simulink library "mcp2515lib"  (R2018b)
settings: Solver=VariableStepAuto  StartTime=0.0  StopTime=10.0  RelTol=1e-3  EnableMultiTasking=on
libraries: $bdroot x33, simulink x26, arduinolib x9, raspberrypilib x9
(part 2 of 2)

== system mcp2515lib/CAN application/CANreceive CE1/readRxBuffer/getDLC ==
  RxBx : Inport
  Bitwise Operator : simulink/Logic and Bit Operations/Bitwise Operator  logicop=AND  UseBitMask=off  NumInputPorts=2  BitMask=bin2dec('11011001')  BitMaskRealWorld=Stored Integer
  MCP_DLC_MASK : Constant  Value=hex2dec('0F')  OutDataTypeStr=uint8
  RxDLC : Selector  IndexMode=Zero-based  InputPortWidth=13  IndexOptions=Index vector (dialog)  Indices=4  OutputSizes=1
  CAN_dlc : Outport
  wires:
  MCP_DLC_MASK/1 -> Bitwise Operator/2
  RxDLC/1 -> Bitwise Operator/1
  RxBx/1 -> RxDLC/1
  Bitwise Operator/1 -> CAN_dlc/1

== system mcp2515lib/CAN application/CANreceive CE1/readRxBuffer/getData ==
  RxBx : Inport
  RxData : Selector  IndexMode=Zero-based  InputPortWidth=13  IndexOptions=Index vector (dialog)  Indices=[5:12]  OutputSizes=1
  CAN_data : Outport
  wires:
  RxData/1 -> CAN_data/1
  RxBx/1 -> RxData/1

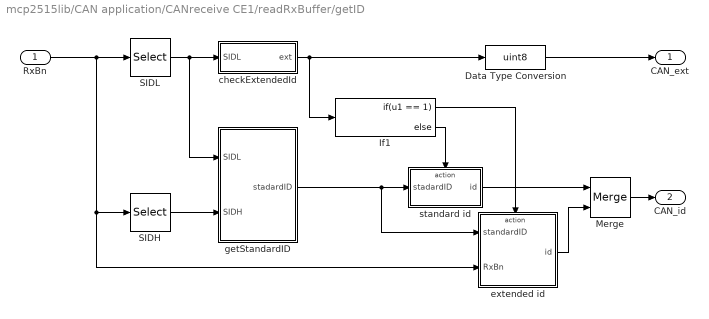
== system mcp2515lib/CAN application/CANreceive CE1/readRxBuffer/getID ==
  RxBn : Inport
  Data Type Conversion : DataTypeConversion  OutDataTypeStr=uint8  RndMeth=Simplest
  If1 : If  IfExpression=u1 == 1
  Merge : Merge
  SIDH : Selector  IndexMode=Zero-based  InputPortWidth=13  IndexOptions=Index vector (dialog)  Indices=0  OutputSizes=1
  SIDL : Selector  IndexMode=Zero-based  InputPortWidth=13  IndexOptions=Index vector (dialog)  Indices=1  OutputSizes=1
  checkExtendedId : Subsystem
  extended id : Subsystem  TreatAsAtomicUnit=on
      settings: RTWSystemCode=Inline
  getStandardID : Subsystem
  standard id : Subsystem  TreatAsAtomicUnit=on
      settings: RTWSystemCode=Inline
  CAN_ext : Outport
  CAN_id : Outport  Port=2
  wires:
  Data Type Conversion/1 -> CAN_ext/1
  checkExtendedId/1(ext) -> If1/1, Data Type Conversion/1
  SIDH/1 -> getStandardID/2(SIDH)
  SIDL/1 -> checkExtendedId/1(SIDL), getStandardID/1(SIDL)
  getStandardID/1(stadardID) -> extended id/1(standardID), standard id/1(stadardID)
  RxBn/1 -> SIDL/1, SIDH/1, extended id/2(RxBn)
  If1/1 -> extended id/Action
  If1/2 -> standard id/Action
  Merge/1 -> CAN_id/1
  extended id/1(id) -> Merge/2
  standard id/1(id) -> Merge/1

== system mcp2515lib/CAN application/CANtransmit/check TxB0/mcp2515_readRegister ==
  In : Inport
  address : Inport  Port=2  OutDataTypeStr=uint8
  Constant : Constant  Value=0  OutDataTypeStr=uint8
  MCP_READ : Constant  Value=3  OutDataTypeStr=uint8
  SPI driver : $bdroot/CAN application/mcp2515 driver/SPI driver  SystemSampleTime=-1
  Selector : Selector  IndexMode=Zero-based  InputPortWidth=3  IndexOptions=Index vector (dialog)  Indices=2  OutputSizes=1
  Vector Concatenate : Concatenate  NumInputs=3
  Out : Outport
  SPI_data : Outport  Port=2
  wires:
  Vector Concatenate/1 -> SPI driver/1
  Selector/1 -> SPI_data/1
  MCP_READ/1 -> Vector Concatenate/1
  In/1 -> Out/1
  Constant/1 -> Vector Concatenate/3
  address/1 -> Vector Concatenate/2
  SPI driver/1 -> Selector/1

== system mcp2515lib/CAN application/CANtransmit/load Tx data/mcp2515_writeTxBuffer ==
  In : Inport
  cmd_load_tx_buff : Inport  Port=2
  data_tx_buff : Inport  Port=3
  SPI driver : $bdroot/CAN application/mcp2515 driver/SPI driver  SystemSampleTime=-1
  Selector1 : Selector  IndexMode=Zero-based  InputPortWidth=14  IndexOptions=Index vector (dialog)  Indices=0  OutputSizes=1
  Temporary buffer : DataStoreWrite  DataStoreName=temp_1byte
  Vector Concatenate : Concatenate
  Out : Outport
  wires:
  Vector Concatenate/1 -> SPI driver/1
  Selector1/1 -> Temporary buffer/1
  cmd_load_tx_buff/1 -> Vector Concatenate/1
  data_tx_buff/1 -> Vector Concatenate/2
  SPI driver/1 -> Selector1/1
  In/1 -> Out/1

== system mcp2515lib/CAN application/CANtransmit/load Tx data/setID ==
  ext : Inport
  id : Inport  Port=2
  Extended ID : Subsystem  TreatAsAtomicUnit=on
  If : If
  Merge : Merge
  Standard ID : Subsystem  TreatAsAtomicUnit=on
  TxBn_ID : Outport
  wires:
  id/1 -> Standard ID/1(id), Extended ID/1(id)
  Merge/1 -> TxBn_ID/1
  Standard ID/1(TxBn_ID) -> Merge/1
  Extended ID/1(TxBn_ID) -> Merge/2
  If/2 -> Standard ID/Action
  If/1 -> Extended ID/Action
  ext/1 -> If/1

== system mcp2515lib/CAN application/CANtransmit/send TxB0/mcp2515_writeRegister ==
  In : Inport
  address : Inport  Port=2  OutDataTypeStr=uint8
  value : Inport  Port=3  OutDataTypeStr=uint8
  MCP_WRITE : Constant  Value=2  OutDataTypeStr=uint8
  SPI driver : $bdroot/CAN application/mcp2515 driver/SPI driver  SystemSampleTime=-1
  Selector : Selector  IndexMode=Zero-based  InputPortWidth=3  IndexOptions=Index vector (dialog)  Indices=0  OutputSizes=1
  Temporary buffer : DataStoreWrite  DataStoreName=temp_1byte
  Vector Concatenate : Concatenate  NumInputs=3
  Out : Outport
  wires:
  MCP_WRITE/1 -> Vector Concatenate/1
  address/1 -> Vector Concatenate/2
  value/1 -> Vector Concatenate/3
  Vector Concatenate/1 -> SPI driver/1
  In/1 -> Out/1
  Selector/1 -> Temporary buffer/1
  SPI driver/1 -> Selector/1

== system mcp2515lib/CAN application/CANtransmit CE1/load Tx data/setID ==
  ext : Inport
  id : Inport  Port=2
  Extended ID : Subsystem  TreatAsAtomicUnit=on
  If : If
  Merge : Merge
  Standard ID : Subsystem  TreatAsAtomicUnit=on
  TxBn_ID : Outport
  wires:
  id/1 -> Standard ID/1(id), Extended ID/1(id)
  Merge/1 -> TxBn_ID/1
  Standard ID/1(TxBn_ID) -> Merge/1
  Extended ID/1(TxBn_ID) -> Merge/2
  If/2 -> Standard ID/Action
  If/1 -> Extended ID/Action
  ext/1 -> If/1

== system mcp2515lib/CAN application/mcp2515 driver/SPI driver/Arduino ==
  SPIdata_In : Inport
  SPI WriteRead : arduinolib/SPI WriteRead  slaveSelectPin_=CSpin  blockPlatform=arduino
      settings: SourceProductName=Simulink Support Package for Arduino Hardware  SourceProductBaseCode=ARDUINO
  SPIdata_Out : Outport
  wires:
  SPIdata_In/1 -> SPI WriteRead/1
  SPI WriteRead/1 -> SPIdata_Out/1

== system mcp2515lib/CAN application/mcp2515 driver/SPI driver/Rapberry Pi ==
  SPIdata_In : Inport
  SPI Master Transfer : raspberrypilib/SPI Master Transfer  BoardProperty=Pi 3 Model B+  SPIModule=uint32(0)  Mode=Master  BusSpeed=1000000  Pin=SPI0_CE0  FirstBitToTransfer=Most significant bit (MSB)  ClockMode=0  BlockFunction=Transfer  RegisterAddress=0  OutputDataType=int8  OutputDataLength=1
      settings: SourceProductName=Simulink Support Package for Raspberry Pi Hardware  SourceProductBaseCode=RASPPI
  SPIdata_Out : Outport
  wires:
  SPIdata_In/1 -> SPI Master Transfer/1
  SPI Master Transfer/1 -> SPIdata_Out/1

== system mcp2515lib/CAN application/mcp2515 driver CE1/SPI driver/Arduino ==
  SPIdata_In : Inport
  SPI WriteRead : arduinolib/SPI WriteRead  slaveSelectPin_=CSpin  blockPlatform=arduino
      settings: SourceProductName=Simulink Support Package for Arduino Hardware  SourceProductBaseCode=ARDUINO
  SPIdata_Out : Outport
  wires:
  SPI WriteRead/1 -> SPIdata_Out/1
  SPIdata_In/1 -> SPI WriteRead/1

== system mcp2515lib/CAN application/mcp2515 driver CE1/SPI driver/Rapberry Pi ==
  SPIdata_In : Inport
  SPI Master Transfer : raspberrypilib/SPI Master Transfer  BoardProperty=Pi 3 Model B+  SPIModule=uint32(0)  Mode=Master  BusSpeed=1000000  Pin=SPI0_CE1  FirstBitToTransfer=Most significant bit (MSB)  ClockMode=0  BlockFunction=Transfer  RegisterAddress=0  OutputDataType=int8  OutputDataLength=1
      settings: SourceProductName=Simulink Support Package for Raspberry Pi Hardware  SourceProductBaseCode=RASPPI
  SPIdata_Out : Outport
  wires:
  SPI Master Transfer/1 -> SPIdata_Out/1
  SPIdata_In/1 -> SPI Master Transfer/1

== system mcp2515lib/CAN application/mcp2515 driver CE1/mcp2515_modifyRegister/SPI driver ==
  SPIdata_In : Inport
  Arduino : Subsystem  TreatAsAtomicUnit=on  VariantControl=Hardware == 1
  Rapberry Pi : Subsystem  TreatAsAtomicUnit=on  VariantControl=Hardware == 2
  SPIdata_Out : Outport

== system mcp2515lib/CAN application/mcp2515 driver CE1/mcp2515_readRegister/SPI driver ==
  SPIdata_In : Inport
  Arduino : Subsystem  TreatAsAtomicUnit=on  VariantControl=Hardware == 1
  Rapberry Pi : Subsystem  TreatAsAtomicUnit=on  VariantControl=Hardware == 2
  SPIdata_Out : Outport

== system mcp2515lib/CAN application/mcp2515 driver CE1/mcp2515_readRxBuffer/SPI driver ==
  SPIdata_In : Inport
  Arduino : Subsystem  TreatAsAtomicUnit=on  VariantControl=Hardware == 1
  Rapberry Pi : Subsystem  TreatAsAtomicUnit=on  VariantControl=Hardware == 2
  SPIdata_Out : Outport

== system mcp2515lib/CAN application/mcp2515 driver CE1/mcp2515_read_RX_STATUS/SPI driver ==
  SPIdata_In : Inport
  Arduino : Subsystem  TreatAsAtomicUnit=on  VariantControl=Hardware == 1
  Rapberry Pi : Subsystem  TreatAsAtomicUnit=on  VariantControl=Hardware == 2
  SPIdata_Out : Outport

== system mcp2515lib/CAN application/mcp2515 driver CE1/mcp2515_reset/SPI driver ==
  SPIdata_In : Inport
  Arduino : Subsystem  TreatAsAtomicUnit=on  VariantControl=Hardware == 1
  Rapberry Pi : Subsystem  TreatAsAtomicUnit=on  VariantControl=Hardware == 2
  SPIdata_Out : Outport

== system mcp2515lib/CAN application/mcp2515 driver CE1/mcp2515_writeRegister/SPI driver ==
  SPIdata_In : Inport
  Arduino : Subsystem  TreatAsAtomicUnit=on  VariantControl=Hardware == 1
  Rapberry Pi : Subsystem  TreatAsAtomicUnit=on  VariantControl=Hardware == 2
  SPIdata_Out : Outport

== system mcp2515lib/CAN application/mcp2515 driver CE1/mcp2515_writeTxBuffer/SPI driver ==
  SPIdata_In : Inport
  Arduino : Subsystem  TreatAsAtomicUnit=on  VariantControl=Hardware == 1
  Rapberry Pi : Subsystem  TreatAsAtomicUnit=on  VariantControl=Hardware == 2
  SPIdata_Out : Outport

== system mcp2515lib/CAN application/CANbegin/setup/changeCANmode(config)/mcp2515_modifyRegister ==
  In : Inport
  address : Inport  Port=2
  mask : Inport  Port=3
  data : Inport  Port=4
  MCP_BITMOD : Constant  Value=5  OutDataTypeStr=uint8
  SPI driver : $bdroot/CAN application/mcp2515 driver/SPI driver  SystemSampleTime=-1
  Selector : Selector  IndexMode=Zero-based  InputPortWidth=4  IndexOptions=Index vector (dialog)  Indices=0  OutputSizes=1
  Temporary buffer : DataStoreWrite  DataStoreName=temp_1byte
  Vector Concatenate : Concatenate  NumInputs=4
  Out : Outport
  wires:
  Vector Concatenate/1 -> SPI driver/1
  Selector/1 -> Temporary buffer/1
  In/1 -> Out/1
  MCP_BITMOD/1 -> Vector Concatenate/1
  mask/1 -> Vector Concatenate/3
  address/1 -> Vector Concatenate/2
  data/1 -> Vector Concatenate/4
  SPI driver/1 -> Selector/1

== system mcp2515lib/CAN application/CANbegin/setup/changeCANmode(normal)/mcp2515_modifyRegister ==
  In : Inport
  address : Inport  Port=2
  mask : Inport  Port=3
  data : Inport  Port=4
  MCP_BITMOD : Constant  Value=5  OutDataTypeStr=uint8
  SPI driver : $bdroot/CAN application/mcp2515 driver/SPI driver  SystemSampleTime=-1
  Selector : Selector  IndexMode=Zero-based  InputPortWidth=4  IndexOptions=Index vector (dialog)  Indices=0  OutputSizes=1
  Temporary buffer : DataStoreWrite  DataStoreName=temp_1byte
  Vector Concatenate : Concatenate  NumInputs=4
  Out : Outport
  wires:
  Vector Concatenate/1 -> SPI driver/1
  Selector/1 -> Temporary buffer/1
  In/1 -> Out/1
  MCP_BITMOD/1 -> Vector Concatenate/1
  mask/1 -> Vector Concatenate/3
  address/1 -> Vector Concatenate/2
  data/1 -> Vector Concatenate/4
  SPI driver/1 -> Selector/1

== system mcp2515lib/CAN application/CANbegin/setup/setCANRxBuffer/mcp2515_writeRegister ==
  In : Inport
  address : Inport  Port=2  OutDataTypeStr=uint8
  value : Inport  Port=3  OutDataTypeStr=uint8
  MCP_WRITE : Constant  Value=2  OutDataTypeStr=uint8
  SPI driver : $bdroot/CAN application/mcp2515 driver/SPI driver  SystemSampleTime=-1
  Selector : Selector  IndexMode=Zero-based  InputPortWidth=3  IndexOptions=Index vector (dialog)  Indices=0  OutputSizes=1
  Temporary buffer : DataStoreWrite  DataStoreName=temp_1byte
  Vector Concatenate : Concatenate  NumInputs=3
  Out : Outport
  wires:
  MCP_WRITE/1 -> Vector Concatenate/1
  address/1 -> Vector Concatenate/2
  value/1 -> Vector Concatenate/3
  Vector Concatenate/1 -> SPI driver/1
  In/1 -> Out/1
  Selector/1 -> Temporary buffer/1
  SPI driver/1 -> Selector/1

== system mcp2515lib/CAN application/CANbegin/setup/setCANRxBuffer/mcp2515_writeRegister1 ==
  In : Inport
  address : Inport  Port=2  OutDataTypeStr=uint8
  value : Inport  Port=3  OutDataTypeStr=uint8
  MCP_WRITE : Constant  Value=2  OutDataTypeStr=uint8
  SPI driver : $bdroot/CAN application/mcp2515 driver/SPI driver  SystemSampleTime=-1
  Selector : Selector  IndexMode=Zero-based  InputPortWidth=3  IndexOptions=Index vector (dialog)  Indices=0  OutputSizes=1
  Temporary buffer : DataStoreWrite  DataStoreName=temp_1byte
  Vector Concatenate : Concatenate  NumInputs=3
  Out : Outport
  wires:
  MCP_WRITE/1 -> Vector Concatenate/1
  address/1 -> Vector Concatenate/2
  value/1 -> Vector Concatenate/3
  Vector Concatenate/1 -> SPI driver/1
  In/1 -> Out/1
  Selector/1 -> Temporary buffer/1
  SPI driver/1 -> Selector/1

== system mcp2515lib/CAN application/CANbegin/setup/setCANspeed/mcp2515_writeRegister1 ==
  In : Inport
  address : Inport  Port=2  OutDataTypeStr=uint8
  value : Inport  Port=3  OutDataTypeStr=uint8
  MCP_WRITE : Constant  Value=2  OutDataTypeStr=uint8
  SPI driver : $bdroot/CAN application/mcp2515 driver/SPI driver  SystemSampleTime=-1
  Selector : Selector  IndexMode=Zero-based  InputPortWidth=3  IndexOptions=Index vector (dialog)  Indices=0  OutputSizes=1
  Temporary buffer : DataStoreWrite  DataStoreName=temp_1byte
  Vector Concatenate : Concatenate  NumInputs=3
  Out : Outport
  wires:
  MCP_WRITE/1 -> Vector Concatenate/1
  address/1 -> Vector Concatenate/2
  value/1 -> Vector Concatenate/3
  Vector Concatenate/1 -> SPI driver/1
  In/1 -> Out/1
  Selector/1 -> Temporary buffer/1
  SPI driver/1 -> Selector/1

== system mcp2515lib/CAN application/CANbegin/setup/setCANspeed/mcp2515_writeRegister2 ==
  In : Inport
  address : Inport  Port=2  OutDataTypeStr=uint8
  value : Inport  Port=3  OutDataTypeStr=uint8
  MCP_WRITE : Constant  Value=2  OutDataTypeStr=uint8
  SPI driver : $bdroot/CAN application/mcp2515 driver/SPI driver  SystemSampleTime=-1
  Selector : Selector  IndexMode=Zero-based  InputPortWidth=3  IndexOptions=Index vector (dialog)  Indices=0  OutputSizes=1
  Temporary buffer : DataStoreWrite  DataStoreName=temp_1byte
  Vector Concatenate : Concatenate  NumInputs=3
  Out : Outport
  wires:
  MCP_WRITE/1 -> Vector Concatenate/1
  address/1 -> Vector Concatenate/2
  value/1 -> Vector Concatenate/3
  Vector Concatenate/1 -> SPI driver/1
  In/1 -> Out/1
  Selector/1 -> Temporary buffer/1
  SPI driver/1 -> Selector/1

== system mcp2515lib/CAN application/CANbegin/setup/setCANspeed/mcp2515_writeRegister3 ==
  In : Inport
  address : Inport  Port=2  OutDataTypeStr=uint8
  value : Inport  Port=3  OutDataTypeStr=uint8
  MCP_WRITE : Constant  Value=2  OutDataTypeStr=uint8
  SPI driver : $bdroot/CAN application/mcp2515 driver/SPI driver  SystemSampleTime=-1
  Selector : Selector  IndexMode=Zero-based  InputPortWidth=3  IndexOptions=Index vector (dialog)  Indices=0  OutputSizes=1
  Temporary buffer : DataStoreWrite  DataStoreName=temp_1byte
  Vector Concatenate : Concatenate  NumInputs=3
  Out : Outport
  wires:
  MCP_WRITE/1 -> Vector Concatenate/1
  address/1 -> Vector Concatenate/2
  value/1 -> Vector Concatenate/3
  Vector Concatenate/1 -> SPI driver/1
  In/1 -> Out/1
  Selector/1 -> Temporary buffer/1
  SPI driver/1 -> Selector/1

== system mcp2515lib/CAN application/CANreceive/readRxBuffer/getID/checkExtendedId ==
  SIDL : Inport
  Bitmask_EXIDE : simulink/Logic and Bit Operations/Bitwise Operator  logicop=AND  UseBitMask=on  BitMask=bin2dec('00001000')  BitMaskRealWorld=Stored Integer
  MCP_TXB_EXIDE_M : Constant  Value=hex2dec('08')  OutDataTypeStr=uint8
  Relational Operator : RelationalOperator  Operator===  OutDataTypeStr=boolean  RndMeth=Nearest
  ext : Outport
  wires:
  SIDL/1 -> Bitmask_EXIDE/1
  Bitmask_EXIDE/1 -> Relational Operator/2
  MCP_TXB_EXIDE_M/1 -> Relational Operator/1
  Relational Operator/1 -> ext/1

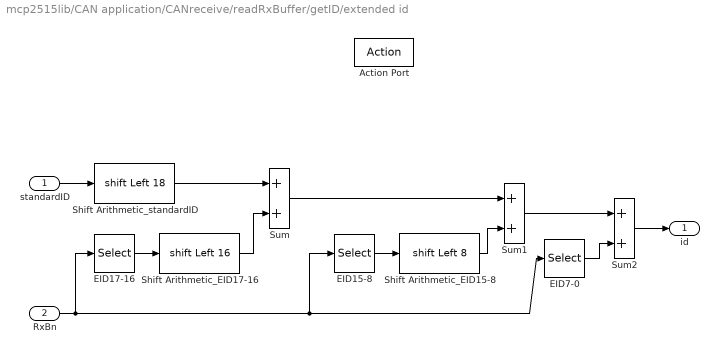
== system mcp2515lib/CAN application/CANreceive/readRxBuffer/getID/extended id ==
  standardID : Inport
  RxBn : Inport  Port=2
  Action Port : ActionPort
  EID15-8 : Selector  IndexMode=Zero-based  InputPortWidth=13  IndexOptions=Index vector (dialog)  Indices=2  OutputSizes=1
  EID17-16 : Selector  IndexMode=Zero-based  InputPortWidth=13  IndexOptions=Index vector (dialog)  Indices=1  OutputSizes=1
  EID7-0 : Selector  IndexMode=Zero-based  InputPortWidth=13  IndexOptions=Index vector (dialog)  Indices=3  OutputSizes=1
  Shift Arithmetic_EID15-8 : ArithShift  BitShiftNumber=8  BitShiftDirection=Left
  Shift Arithmetic_EID17-16 : ArithShift  BitShiftNumber=16  BitShiftDirection=Left
  Shift Arithmetic_standardID : ArithShift  BitShiftNumber=18  BitShiftDirection=Left
  Sum : Sum
  Sum1 : Sum
  Sum2 : Sum
  id : Outport
  wires:
  EID7-0/1 -> Sum2/2
  RxBn/1 -> EID17-16/1, EID15-8/1, EID7-0/1
  Sum1/1 -> Sum2/1
  EID15-8/1 -> Shift Arithmetic_EID15-8/1
  Shift Arithmetic_EID15-8/1 -> Sum1/2
  Sum/1 -> Sum1/1
  Shift Arithmetic_EID17-16/1 -> Sum/2
  EID17-16/1 -> Shift Arithmetic_EID17-16/1
  Shift Arithmetic_standardID/1 -> Sum/1
  standardID/1 -> Shift Arithmetic_standardID/1
  Sum2/1 -> id/1

== system mcp2515lib/CAN application/CANreceive/readRxBuffer/getID/getStandardID ==
  SIDL : Inport
  SIDH : Inport  Port=2
  Bitmask_SID2-0 : simulink/Logic and Bit Operations/Bitwise Operator  logicop=AND  UseBitMask=on  BitMask=bin2dec('11100000')  BitMaskRealWorld=Stored Integer
  Data Type Conversion : DataTypeConversion  OutDataTypeStr=uint32
  Shift Arithmetic_SID10-3 : ArithShift  BitShiftNumber=3  BitShiftDirection=Left
  Shift Arithmetic_SID2-0 : ArithShift  BitShiftNumber=5  BitShiftDirection=Right
  Sum1 : Sum
  stadardID : Outport
  wires:
  Data Type Conversion/1 -> Shift Arithmetic_SID10-3/1
  Bitmask_SID2-0/1 -> Shift Arithmetic_SID2-0/1
  SIDH/1 -> Data Type Conversion/1
  SIDL/1 -> Bitmask_SID2-0/1
  Shift Arithmetic_SID10-3/1 -> Sum1/2
  Shift Arithmetic_SID2-0/1 -> Sum1/1
  Sum1/1 -> stadardID/1

== system mcp2515lib/CAN application/CANreceive/readRxBuffer/getID/standard id ==
  stadardID : Inport
  Action Port : ActionPort
  id : Outport
  wires:
  stadardID/1 -> id/1

== system mcp2515lib/CAN application/CANreceive CE1/readRxBuffer/getID/checkExtendedId ==
  SIDL : Inport
  Bitmask_EXIDE : simulink/Logic and Bit Operations/Bitwise Operator  logicop=AND  UseBitMask=on  BitMask=bin2dec('00001000')  BitMaskRealWorld=Stored Integer
  MCP_TXB_EXIDE_M : Constant  Value=hex2dec('08')  OutDataTypeStr=uint8
  Relational Operator : RelationalOperator  Operator===  OutDataTypeStr=boolean  RndMeth=Nearest
  ext : Outport
  wires:
  SIDL/1 -> Bitmask_EXIDE/1
  Bitmask_EXIDE/1 -> Relational Operator/2
  MCP_TXB_EXIDE_M/1 -> Relational Operator/1
  Relational Operator/1 -> ext/1

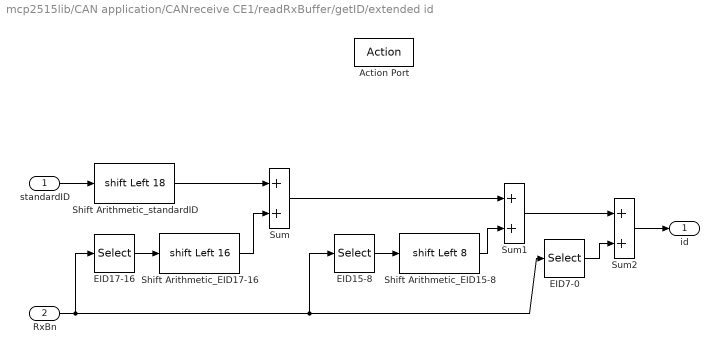
== system mcp2515lib/CAN application/CANreceive CE1/readRxBuffer/getID/extended id ==
  standardID : Inport
  RxBn : Inport  Port=2
  Action Port : ActionPort
  EID15-8 : Selector  IndexMode=Zero-based  InputPortWidth=13  IndexOptions=Index vector (dialog)  Indices=2  OutputSizes=1
  EID17-16 : Selector  IndexMode=Zero-based  InputPortWidth=13  IndexOptions=Index vector (dialog)  Indices=1  OutputSizes=1
  EID7-0 : Selector  IndexMode=Zero-based  InputPortWidth=13  IndexOptions=Index vector (dialog)  Indices=3  OutputSizes=1
  Shift Arithmetic_EID15-8 : ArithShift  BitShiftNumber=8  BitShiftDirection=Left
  Shift Arithmetic_EID17-16 : ArithShift  BitShiftNumber=16  BitShiftDirection=Left
  Shift Arithmetic_standardID : ArithShift  BitShiftNumber=18  BitShiftDirection=Left
  Sum : Sum
  Sum1 : Sum
  Sum2 : Sum
  id : Outport
  wires:
  EID7-0/1 -> Sum2/2
  RxBn/1 -> EID17-16/1, EID15-8/1, EID7-0/1
  Sum1/1 -> Sum2/1
  EID15-8/1 -> Shift Arithmetic_EID15-8/1
  Shift Arithmetic_EID15-8/1 -> Sum1/2
  Sum/1 -> Sum1/1
  Shift Arithmetic_EID17-16/1 -> Sum/2
  EID17-16/1 -> Shift Arithmetic_EID17-16/1
  Shift Arithmetic_standardID/1 -> Sum/1
  standardID/1 -> Shift Arithmetic_standardID/1
  Sum2/1 -> id/1

== system mcp2515lib/CAN application/CANreceive CE1/readRxBuffer/getID/getStandardID ==
  SIDL : Inport
  SIDH : Inport  Port=2
  Bitmask_SID2-0 : simulink/Logic and Bit Operations/Bitwise Operator  logicop=AND  UseBitMask=on  BitMask=bin2dec('11100000')  BitMaskRealWorld=Stored Integer
  Data Type Conversion : DataTypeConversion  OutDataTypeStr=uint32
  Shift Arithmetic_SID10-3 : ArithShift  BitShiftNumber=3  BitShiftDirection=Left
  Shift Arithmetic_SID2-0 : ArithShift  BitShiftNumber=5  BitShiftDirection=Right
  Sum1 : Sum
  stadardID : Outport
  wires:
  Data Type Conversion/1 -> Shift Arithmetic_SID10-3/1
  Bitmask_SID2-0/1 -> Shift Arithmetic_SID2-0/1
  SIDH/1 -> Data Type Conversion/1
  SIDL/1 -> Bitmask_SID2-0/1
  Shift Arithmetic_SID10-3/1 -> Sum1/2
  Shift Arithmetic_SID2-0/1 -> Sum1/1
  Sum1/1 -> stadardID/1

== system mcp2515lib/CAN application/CANreceive CE1/readRxBuffer/getID/standard id ==
  stadardID : Inport
  Action Port : ActionPort
  id : Outport
  wires:
  stadardID/1 -> id/1

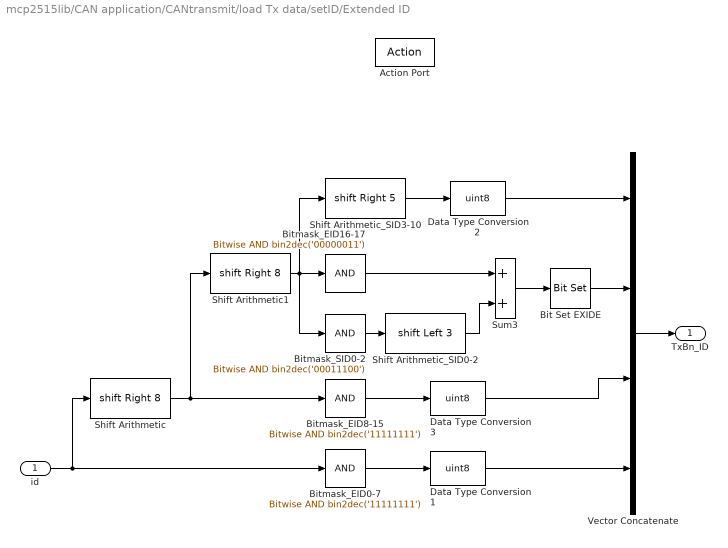
== system mcp2515lib/CAN application/CANtransmit/load Tx data/setID/Extended ID ==
  id : Inport
  Action Port : ActionPort
  Bit Set EXIDE : simulink/Logic and Bit Operations/Bit Set  iBit=3
      settings: SourceProductName=Simulink  SourceProductBaseCode=SL
  Bitmask_EID0-7 : simulink/Logic and Bit Operations/Bitwise Operator  logicop=AND  UseBitMask=on  BitMask=bin2dec('11111111')  BitMaskRealWorld=Stored Integer
  Bitmask_EID16-17 : simulink/Logic and Bit Operations/Bitwise Operator  logicop=AND  UseBitMask=on  BitMask=bin2dec('00000011')  BitMaskRealWorld=Stored Integer
  Bitmask_EID8-15 : simulink/Logic and Bit Operations/Bitwise Operator  logicop=AND  UseBitMask=on  BitMask=bin2dec('11111111')  BitMaskRealWorld=Stored Integer
  Bitmask_SID0-2 : simulink/Logic and Bit Operations/Bitwise Operator  logicop=AND  UseBitMask=on  BitMask=bin2dec('00011100')  BitMaskRealWorld=Stored Integer
  Data Type Conversion1 : DataTypeConversion  OutDataTypeStr=uint8  RndMeth=Simplest
  Data Type Conversion2 : DataTypeConversion  OutDataTypeStr=uint8  RndMeth=Simplest
  Data Type Conversion3 : DataTypeConversion  OutDataTypeStr=uint8  RndMeth=Simplest
  Shift Arithmetic : ArithShift  BitShiftNumber=8  BitShiftDirection=Right
  Shift Arithmetic1 : ArithShift  BitShiftNumber=8  BitShiftDirection=Right
  Shift Arithmetic_SID0-2 : ArithShift  BitShiftNumber=3  BitShiftDirection=Left
  Shift Arithmetic_SID3-10 : ArithShift  BitShiftNumber=5  BitShiftDirection=Right
  Sum3 : Sum  OutDataTypeStr=uint8
  Vector Concatenate : Concatenate  NumInputs=4
  TxBn_ID : Outport
  wires:
  Data Type Conversion2/1 -> Vector Concatenate/1
  Shift Arithmetic_SID3-10/1 -> Data Type Conversion2/1
  Bit Set EXIDE/1 -> Vector Concatenate/2
  Shift Arithmetic_SID0-2/1 -> Sum3/2
  Bitmask_SID0-2/1 -> Shift Arithmetic_SID0-2/1
  Bitmask_EID16-17/1 -> Sum3/1
  Sum3/1 -> Bit Set EXIDE/1
  Shift Arithmetic1/1 -> Bitmask_EID16-17/1, Bitmask_SID0-2/1, Shift Arithmetic_SID3-10/1
  Data Type Conversion3/1 -> Vector Concatenate/3
  Bitmask_EID8-15/1 -> Data Type Conversion3/1
  Shift Arithmetic/1 -> Bitmask_EID8-15/1, Shift Arithmetic1/1
  Data Type Conversion1/1 -> Vector Concatenate/4
  Bitmask_EID0-7/1 -> Data Type Conversion1/1
  id/1 -> Bitmask_EID0-7/1, Shift Arithmetic/1
  Vector Concatenate/1 -> TxBn_ID/1

== system mcp2515lib/CAN application/CANtransmit/load Tx data/setID/Standard ID ==
  id : Inport
  Action Port : ActionPort
  Vector Concatenate : Concatenate  NumInputs=4
  convert_ID : Subsystem  TreatAsAtomicUnit=on
  no data : Constant  Value=0  OutDataTypeStr=uint8
  TxBn_ID : Outport
  wires:
  convert_ID/1(SIDH) -> Vector Concatenate/1
  id/1 -> convert_ID/1(id)
  convert_ID/2(SIDL) -> Vector Concatenate/2
  no data/1 -> Vector Concatenate/4, Vector Concatenate/3
  Vector Concatenate/1 -> TxBn_ID/1

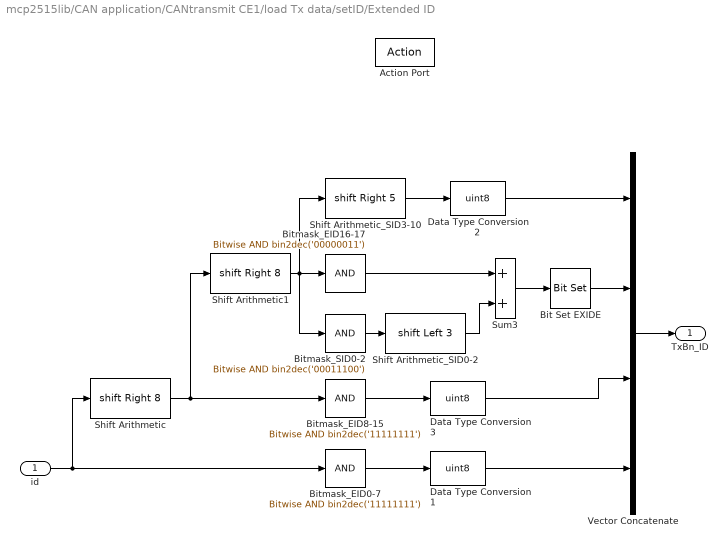
== system mcp2515lib/CAN application/CANtransmit CE1/load Tx data/setID/Extended ID ==
  id : Inport
  Action Port : ActionPort
  Bit Set EXIDE : simulink/Logic and Bit Operations/Bit Set  iBit=3
      settings: SourceProductName=Simulink  SourceProductBaseCode=SL
  Bitmask_EID0-7 : simulink/Logic and Bit Operations/Bitwise Operator  logicop=AND  UseBitMask=on  BitMask=bin2dec('11111111')  BitMaskRealWorld=Stored Integer
  Bitmask_EID16-17 : simulink/Logic and Bit Operations/Bitwise Operator  logicop=AND  UseBitMask=on  BitMask=bin2dec('00000011')  BitMaskRealWorld=Stored Integer
  Bitmask_EID8-15 : simulink/Logic and Bit Operations/Bitwise Operator  logicop=AND  UseBitMask=on  BitMask=bin2dec('11111111')  BitMaskRealWorld=Stored Integer
  Bitmask_SID0-2 : simulink/Logic and Bit Operations/Bitwise Operator  logicop=AND  UseBitMask=on  BitMask=bin2dec('00011100')  BitMaskRealWorld=Stored Integer
  Data Type Conversion1 : DataTypeConversion  OutDataTypeStr=uint8  RndMeth=Simplest
  Data Type Conversion2 : DataTypeConversion  OutDataTypeStr=uint8  RndMeth=Simplest
  Data Type Conversion3 : DataTypeConversion  OutDataTypeStr=uint8  RndMeth=Simplest
  Shift Arithmetic : ArithShift  BitShiftNumber=8  BitShiftDirection=Right
  Shift Arithmetic1 : ArithShift  BitShiftNumber=8  BitShiftDirection=Right
  Shift Arithmetic_SID0-2 : ArithShift  BitShiftNumber=3  BitShiftDirection=Left
  Shift Arithmetic_SID3-10 : ArithShift  BitShiftNumber=5  BitShiftDirection=Right
  Sum3 : Sum  OutDataTypeStr=uint8
  Vector Concatenate : Concatenate  NumInputs=4
  TxBn_ID : Outport
  wires:
  Data Type Conversion2/1 -> Vector Concatenate/1
  Shift Arithmetic_SID3-10/1 -> Data Type Conversion2/1
  Bit Set EXIDE/1 -> Vector Concatenate/2
  Shift Arithmetic_SID0-2/1 -> Sum3/2
  Bitmask_SID0-2/1 -> Shift Arithmetic_SID0-2/1
  Bitmask_EID16-17/1 -> Sum3/1
  Sum3/1 -> Bit Set EXIDE/1
  Shift Arithmetic1/1 -> Bitmask_EID16-17/1, Bitmask_SID0-2/1, Shift Arithmetic_SID3-10/1
  Data Type Conversion3/1 -> Vector Concatenate/3
  Bitmask_EID8-15/1 -> Data Type Conversion3/1
  Shift Arithmetic/1 -> Bitmask_EID8-15/1, Shift Arithmetic1/1
  Data Type Conversion1/1 -> Vector Concatenate/4
  Bitmask_EID0-7/1 -> Data Type Conversion1/1
  id/1 -> Bitmask_EID0-7/1, Shift Arithmetic/1
  Vector Concatenate/1 -> TxBn_ID/1

== system mcp2515lib/CAN application/CANtransmit CE1/load Tx data/setID/Standard ID ==
  id : Inport
  Action Port : ActionPort
  Vector Concatenate : Concatenate  NumInputs=4
  convert_ID : Subsystem  TreatAsAtomicUnit=on
  no data : Constant  Value=0  OutDataTypeStr=uint8
  TxBn_ID : Outport
  wires:
  convert_ID/1(SIDH) -> Vector Concatenate/1
  id/1 -> convert_ID/1(id)
  convert_ID/2(SIDL) -> Vector Concatenate/2
  no data/1 -> Vector Concatenate/4, Vector Concatenate/3
  Vector Concatenate/1 -> TxBn_ID/1

== system mcp2515lib/CAN application/mcp2515 driver CE1/mcp2515_modifyRegister/SPI driver/Arduino ==
  SPIdata_In : Inport
  SPI WriteRead : arduinolib/SPI WriteRead  slaveSelectPin_=CSpin  blockPlatform=arduino
      settings: SourceProductName=Simulink Support Package for Arduino Hardware  SourceProductBaseCode=ARDUINO
  SPIdata_Out : Outport
  wires:
  SPI WriteRead/1 -> SPIdata_Out/1
  SPIdata_In/1 -> SPI WriteRead/1

== system mcp2515lib/CAN application/mcp2515 driver CE1/mcp2515_modifyRegister/SPI driver/Rapberry Pi ==
  SPIdata_In : Inport
  SPI Master Transfer : raspberrypilib/SPI Master Transfer  BoardProperty=Pi 3 Model B+  SPIModule=uint32(0)  Mode=Master  BusSpeed=1000000  Pin=SPI0_CE1  FirstBitToTransfer=Most significant bit (MSB)  ClockMode=0  BlockFunction=Transfer  RegisterAddress=0  OutputDataType=int8  OutputDataLength=1
      settings: SourceProductName=Simulink Support Package for Raspberry Pi Hardware  SourceProductBaseCode=RASPPI
  SPIdata_Out : Outport
  wires:
  SPI Master Transfer/1 -> SPIdata_Out/1
  SPIdata_In/1 -> SPI Master Transfer/1

== system mcp2515lib/CAN application/mcp2515 driver CE1/mcp2515_readRegister/SPI driver/Arduino ==
  SPIdata_In : Inport
  SPI WriteRead : arduinolib/SPI WriteRead  slaveSelectPin_=CSpin  blockPlatform=arduino
      settings: SourceProductName=Simulink Support Package for Arduino Hardware  SourceProductBaseCode=ARDUINO
  SPIdata_Out : Outport
  wires:
  SPI WriteRead/1 -> SPIdata_Out/1
  SPIdata_In/1 -> SPI WriteRead/1

== system mcp2515lib/CAN application/mcp2515 driver CE1/mcp2515_readRegister/SPI driver/Rapberry Pi ==
  SPIdata_In : Inport
  SPI Master Transfer : raspberrypilib/SPI Master Transfer  BoardProperty=Pi 3 Model B+  SPIModule=uint32(0)  Mode=Master  BusSpeed=1000000  Pin=SPI0_CE1  FirstBitToTransfer=Most significant bit (MSB)  ClockMode=0  BlockFunction=Transfer  RegisterAddress=0  OutputDataType=int8  OutputDataLength=1
      settings: SourceProductName=Simulink Support Package for Raspberry Pi Hardware  SourceProductBaseCode=RASPPI
  SPIdata_Out : Outport
  wires:
  SPI Master Transfer/1 -> SPIdata_Out/1
  SPIdata_In/1 -> SPI Master Transfer/1

== system mcp2515lib/CAN application/mcp2515 driver CE1/mcp2515_readRxBuffer/SPI driver/Arduino ==
  SPIdata_In : Inport
  SPI WriteRead : arduinolib/SPI WriteRead  slaveSelectPin_=CSpin  blockPlatform=arduino
      settings: SourceProductName=Simulink Support Package for Arduino Hardware  SourceProductBaseCode=ARDUINO
  SPIdata_Out : Outport
  wires:
  SPI WriteRead/1 -> SPIdata_Out/1
  SPIdata_In/1 -> SPI WriteRead/1

== system mcp2515lib/CAN application/mcp2515 driver CE1/mcp2515_readRxBuffer/SPI driver/Rapberry Pi ==
  SPIdata_In : Inport
  SPI Master Transfer : raspberrypilib/SPI Master Transfer  BoardProperty=Pi 3 Model B+  SPIModule=uint32(0)  Mode=Master  BusSpeed=1000000  Pin=SPI0_CE1  FirstBitToTransfer=Most significant bit (MSB)  ClockMode=0  BlockFunction=Transfer  RegisterAddress=0  OutputDataType=int8  OutputDataLength=1
      settings: SourceProductName=Simulink Support Package for Raspberry Pi Hardware  SourceProductBaseCode=RASPPI
  SPIdata_Out : Outport
  wires:
  SPI Master Transfer/1 -> SPIdata_Out/1
  SPIdata_In/1 -> SPI Master Transfer/1

== system mcp2515lib/CAN application/mcp2515 driver CE1/mcp2515_read_RX_STATUS/SPI driver/Arduino ==
  SPIdata_In : Inport
  SPI WriteRead : arduinolib/SPI WriteRead  slaveSelectPin_=CSpin  blockPlatform=arduino
      settings: SourceProductName=Simulink Support Package for Arduino Hardware  SourceProductBaseCode=ARDUINO
  SPIdata_Out : Outport
  wires:
  SPI WriteRead/1 -> SPIdata_Out/1
  SPIdata_In/1 -> SPI WriteRead/1

== system mcp2515lib/CAN application/mcp2515 driver CE1/mcp2515_read_RX_STATUS/SPI driver/Rapberry Pi ==
  SPIdata_In : Inport
  SPI Master Transfer : raspberrypilib/SPI Master Transfer  BoardProperty=Pi 3 Model B+  SPIModule=uint32(0)  Mode=Master  BusSpeed=1000000  Pin=SPI0_CE1  FirstBitToTransfer=Most significant bit (MSB)  ClockMode=0  BlockFunction=Transfer  RegisterAddress=0  OutputDataType=int8  OutputDataLength=1
      settings: SourceProductName=Simulink Support Package for Raspberry Pi Hardware  SourceProductBaseCode=RASPPI
  SPIdata_Out : Outport
  wires:
  SPI Master Transfer/1 -> SPIdata_Out/1
  SPIdata_In/1 -> SPI Master Transfer/1

== system mcp2515lib/CAN application/mcp2515 driver CE1/mcp2515_reset/SPI driver/Arduino ==
  SPIdata_In : Inport
  SPI WriteRead : arduinolib/SPI WriteRead  slaveSelectPin_=CSpin  blockPlatform=arduino
      settings: SourceProductName=Simulink Support Package for Arduino Hardware  SourceProductBaseCode=ARDUINO
  SPIdata_Out : Outport
  wires:
  SPI WriteRead/1 -> SPIdata_Out/1
  SPIdata_In/1 -> SPI WriteRead/1

== system mcp2515lib/CAN application/mcp2515 driver CE1/mcp2515_reset/SPI driver/Rapberry Pi ==
  SPIdata_In : Inport
  SPI Master Transfer : raspberrypilib/SPI Master Transfer  BoardProperty=Pi 3 Model B+  SPIModule=uint32(0)  Mode=Master  BusSpeed=1000000  Pin=SPI0_CE1  FirstBitToTransfer=Most significant bit (MSB)  ClockMode=0  BlockFunction=Transfer  RegisterAddress=0  OutputDataType=int8  OutputDataLength=1
      settings: SourceProductName=Simulink Support Package for Raspberry Pi Hardware  SourceProductBaseCode=RASPPI
  SPIdata_Out : Outport
  wires:
  SPI Master Transfer/1 -> SPIdata_Out/1
  SPIdata_In/1 -> SPI Master Transfer/1

== system mcp2515lib/CAN application/mcp2515 driver CE1/mcp2515_writeRegister/SPI driver/Arduino ==
  SPIdata_In : Inport
  SPI WriteRead : arduinolib/SPI WriteRead  slaveSelectPin_=CSpin  blockPlatform=arduino
      settings: SourceProductName=Simulink Support Package for Arduino Hardware  SourceProductBaseCode=ARDUINO
  SPIdata_Out : Outport
  wires:
  SPI WriteRead/1 -> SPIdata_Out/1
  SPIdata_In/1 -> SPI WriteRead/1

== system mcp2515lib/CAN application/mcp2515 driver CE1/mcp2515_writeRegister/SPI driver/Rapberry Pi ==
  SPIdata_In : Inport
  SPI Master Transfer : raspberrypilib/SPI Master Transfer  BoardProperty=Pi 3 Model B+  SPIModule=uint32(0)  Mode=Master  BusSpeed=1000000  Pin=SPI0_CE1  FirstBitToTransfer=Most significant bit (MSB)  ClockMode=0  BlockFunction=Transfer  RegisterAddress=0  OutputDataType=int8  OutputDataLength=1
      settings: SourceProductName=Simulink Support Package for Raspberry Pi Hardware  SourceProductBaseCode=RASPPI
  SPIdata_Out : Outport
  wires:
  SPI Master Transfer/1 -> SPIdata_Out/1
  SPIdata_In/1 -> SPI Master Transfer/1

== system mcp2515lib/CAN application/mcp2515 driver CE1/mcp2515_writeTxBuffer/SPI driver/Arduino ==
  SPIdata_In : Inport
  SPI WriteRead : arduinolib/SPI WriteRead  slaveSelectPin_=CSpin  blockPlatform=arduino
      settings: SourceProductName=Simulink Support Package for Arduino Hardware  SourceProductBaseCode=ARDUINO
  SPIdata_Out : Outport
  wires:
  SPI WriteRead/1 -> SPIdata_Out/1
  SPIdata_In/1 -> SPI WriteRead/1

== system mcp2515lib/CAN application/mcp2515 driver CE1/mcp2515_writeTxBuffer/SPI driver/Rapberry Pi ==
  SPIdata_In : Inport
  SPI Master Transfer : raspberrypilib/SPI Master Transfer  BoardProperty=Pi 3 Model B+  SPIModule=uint32(0)  Mode=Master  BusSpeed=1000000  Pin=SPI0_CE1  FirstBitToTransfer=Most significant bit (MSB)  ClockMode=0  BlockFunction=Transfer  RegisterAddress=0  OutputDataType=int8  OutputDataLength=1
      settings: SourceProductName=Simulink Support Package for Raspberry Pi Hardware  SourceProductBaseCode=RASPPI
  SPIdata_Out : Outport
  wires:
  SPI Master Transfer/1 -> SPIdata_Out/1
  SPIdata_In/1 -> SPI Master Transfer/1

== system mcp2515lib/CAN application/CANtransmit/load Tx data/setID/Standard ID/convert_ID ==
  id : Inport
  Bitmask_SID0-10 : simulink/Logic and Bit Operations/Bitwise Operator  logicop=AND  UseBitMask=on  BitMask=bin2dec('0000011111111111')  BitMaskRealWorld=Stored Integer
  Bitmask_SID0-2 : simulink/Logic and Bit Operations/Bitwise Operator  logicop=AND  UseBitMask=on  BitMask=bin2dec('0000000011100000')  BitMaskRealWorld=Stored Integer
  Data Type Conversion1 : DataTypeConversion  OutDataTypeStr=uint8  RndMeth=Simplest
  Data Type Conversion2 : DataTypeConversion  OutDataTypeStr=uint8  RndMeth=Simplest
  Shift Arithmetic1 : ArithShift  BitShiftNumber=3  BitShiftDirection=Right
  Shift Arithmetic2 : ArithShift  BitShiftNumber=5  BitShiftDirection=Left
  SIDH : Outport
  SIDL : Outport  Port=2
  wires:
  Bitmask_SID0-2/1 -> Data Type Conversion2/1
  id/1 -> Bitmask_SID0-10/1
  Shift Arithmetic2/1 -> Bitmask_SID0-2/1
  Data Type Conversion2/1 -> SIDL/1
  Bitmask_SID0-10/1 -> Shift Arithmetic1/1, Shift Arithmetic2/1
  Data Type Conversion1/1 -> SIDH/1
  Shift Arithmetic1/1 -> Data Type Conversion1/1

== system mcp2515lib/CAN application/CANtransmit CE1/load Tx data/setID/Standard ID/convert_ID ==
  id : Inport
  Bitmask_SID0-10 : simulink/Logic and Bit Operations/Bitwise Operator  logicop=AND  UseBitMask=on  BitMask=bin2dec('0000011111111111')  BitMaskRealWorld=Stored Integer
  Bitmask_SID0-2 : simulink/Logic and Bit Operations/Bitwise Operator  logicop=AND  UseBitMask=on  BitMask=bin2dec('0000000011100000')  BitMaskRealWorld=Stored Integer
  Data Type Conversion1 : DataTypeConversion  OutDataTypeStr=uint8  RndMeth=Simplest
  Data Type Conversion2 : DataTypeConversion  OutDataTypeStr=uint8  RndMeth=Simplest
  Shift Arithmetic1 : ArithShift  BitShiftNumber=3  BitShiftDirection=Right
  Shift Arithmetic2 : ArithShift  BitShiftNumber=5  BitShiftDirection=Left
  SIDH : Outport
  SIDL : Outport  Port=2
  wires:
  Bitmask_SID0-2/1 -> Data Type Conversion2/1
  id/1 -> Bitmask_SID0-10/1
  Shift Arithmetic2/1 -> Bitmask_SID0-2/1
  Data Type Conversion2/1 -> SIDL/1
  Bitmask_SID0-10/1 -> Shift Arithmetic1/1, Shift Arithmetic2/1
  Data Type Conversion1/1 -> SIDH/1
  Shift Arithmetic1/1 -> Data Type Conversion1/1
